simulink model "R2_and_P2_Calculation"  (R2024a)
settings: Solver=VariableStepAuto  StartTime=0.0  StopTime=10.0  RelTol=1e-3
settings Model: Creator=ACER  LastModifiedBy=ACER

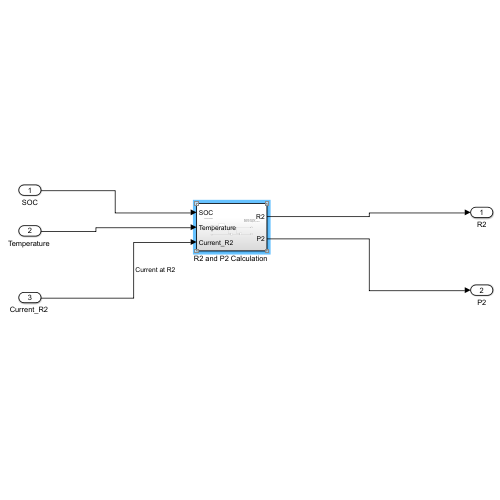
[thumbnail: Simulink's stored preview of the top-level diagram]
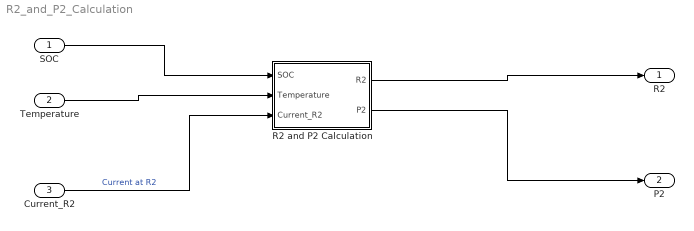
== system R2_and_P2_Calculation ==
  SOC : Inport
  "Temperature " : Inport  Port=2
  "Current_R2 " : Inport  Port=3
  "R2 and P2 Calculation " : Subsystem
  R2 : Outport
  P2 : Outport  Port=2
  wires:
  SOC/1 -> "R2 and P2 Calculation "/1(SOC)
  "Temperature "/1 -> "R2 and P2 Calculation "/2("Temperature ")
  "Current_R2 "/1 -> "R2 and P2 Calculation "/3("Current_R2 ")  "Current at R2"
  "R2 and P2 Calculation "/1(R2) -> R2/1
  "R2 and P2 Calculation "/2(P2) -> P2/1

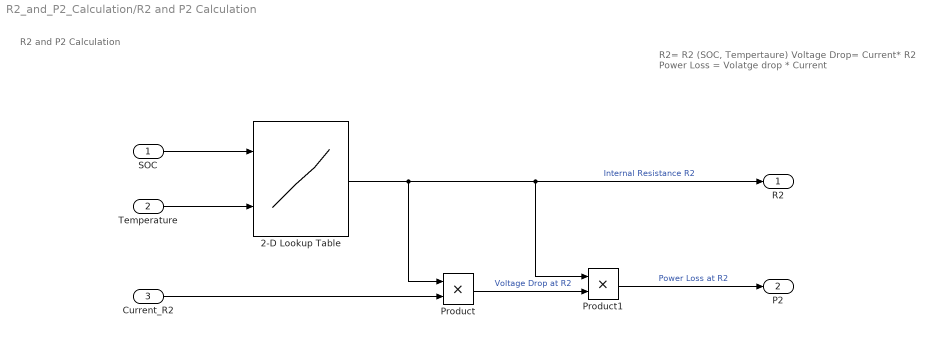
== system R2_and_P2_Calculation/R2 and P2 Calculation  ==
  note: R2 and P2 Calculation
  note: R2= R2 (SOC, Tempertaure)
      | Voltage Drop= Current* R2
      | Power Loss = Volatge drop * Current
  SOC : Inport
  "Temperature " : Inport  Port=2
  "Current_R2 " : Inport  Port=3
  2-D Lookup Table : Lookup_n-D  BreakpointsForDimension1=[1:3]  BreakpointsForDimension2=[1:3]  InternalRulePriority=Speed  RndMeth=Simplest
      settings: InputPortMap=u0,u1
  Product : Product
  Product1 : Product
  R2 : Outport
  P2 : Outport  Port=2
  wires:
  2-D Lookup Table/1 -> R2/1, Product1/1, Product/1  "Internal Resistance R2"
  Product1/1 -> P2/1  "Power Loss at R2"
  "Temperature "/1 -> 2-D Lookup Table/2
  Product/1 -> Product1/2  "Voltage Drop at R2"
  SOC/1 -> 2-D Lookup Table/1
  "Current_R2 "/1 -> Product/2
